simulink model "FIR_32tap_HIL"  (Simulink 7.0)
settings: Solver=FixedStepDiscrete  StartTime=0.0  StopTime=1024*sample_time  RelTol=1e-3
PreLoadFcn:
  | FIR_32tap_setup
InitFcn:
  | %% DSPBuilder Start
  | alt_dspbuilder_update_model(bdroot)
  | %% DSPBuilder End
undefined symbols (not defined in the file): get, sample_time
libraries: allblocks_alteradspbuilder2 x8, dspsnks4 x2, simulink x1
settings Model: Creator=davlin  LastModifiedBy=davlin
settings DebuggingCC: SaveWithParameterizedLinksMsg=none
settings GRTTargetCC: TargetFcnLib=ansi_tfl_tmw.mat

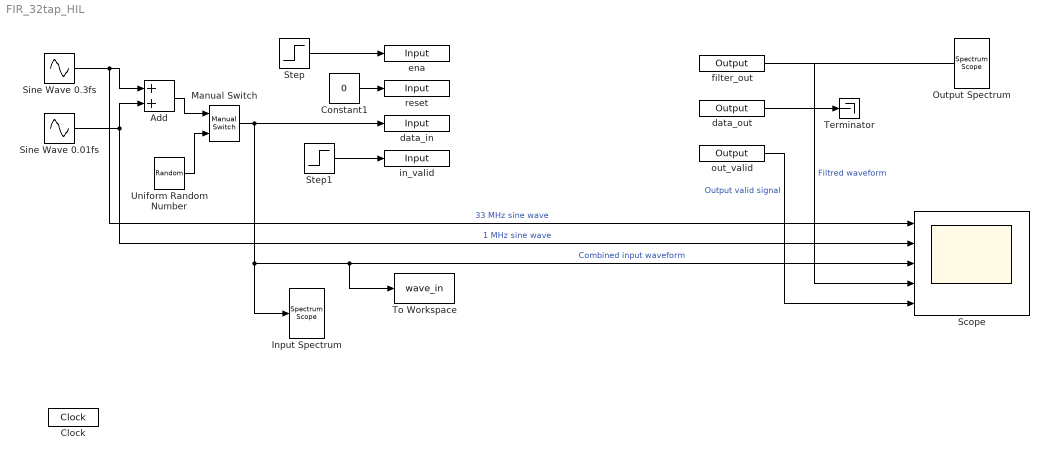
== system FIR_32tap_HIL ==
  Add : Sum  OutDataType=sfix(16)  OutScaling=2^-10
  Clock : allblocks_alteradspbuilder2/Clock  ClockPeriod=clock_period  ClockPeriodUnit=ns  SampleTime=sample_time  SimulationStartCycle=5  PhaseOffset=0  Reset=aclr  ResetType=Active Low  Export=off
  Constant1 : Constant  Value=0  OutDataType=sfix(16)  OutScaling=2^0  SampleTime=sample_time
  Input Spectrum : dspsnks4/Spectrum Scope  DialogController=dspdialog.SpectrumScope  DialogControllerArgs=DataTag0  SystemSampleTime=-1  ScopeProperties=on  Domain=Frequency  HorizSpan=1  UseBuffer=on  BufferSize=128  Overlap=64  inpFftLenInherit=off  FFTlength=128  numAvg=2  DisplayProperties=off  AxisGrid=on  Memory=off  FrameNumber=on  AxisLegend=off  AxisZoom=off  OpenScopeAtSimStart=on  OpenScopeImmediately=off  FigPos=get(0,'defaultfigureposition')  AxisProperties=off  XUnits=Hertz  XRange=[0...Fs/2]  InheritXIncr=on  XIncr=1.0  XLabel=Samples  XLimit=Auto  YUnits=dB  XMax=1  XMin=0  YLabel=Magnitude-squared, dB  LineProperties=off  wintypeSpecScope=Kaiser  RsSpecScope=50  betaSpecScope=5  winsampSpecScope=Periodic
      settings: YMin=7.87541679161896  YMax=68.8425321075722
  Manual Switch : simulink/Signal Routing/Manual Switch  SystemSampleTime=-1  sw=1  action=0  varsize=off
  Output Spectrum : dspsnks4/Spectrum Scope  DialogController=dspdialog.SpectrumScope  DialogControllerArgs=DataTag1  SystemSampleTime=-1  ScopeProperties=on  Domain=Frequency  HorizSpan=1  UseBuffer=on  BufferSize=128  Overlap=64  inpFftLenInherit=off  FFTlength=128  numAvg=2  DisplayProperties=off  AxisGrid=on  Memory=off  FrameNumber=on  AxisLegend=off  AxisZoom=off  OpenScopeAtSimStart=on  OpenScopeImmediately=off  FigPos=get(0,'defaultfigureposition')  AxisProperties=off  XUnits=Hertz  XRange=[0...Fs/2]  InheritXIncr=on  XIncr=1.0  XLabel=Samples  XLimit=Auto  YUnits=dB  XMax=1  XMin=0  YLabel=Magnitude-squared, dB  LineProperties=off  wintypeSpecScope=Kaiser  RsSpecScope=50  betaSpecScope=5  winsampSpecScope=Periodic
      settings: YMin=64.9503892288853  YMax=135.181542756045
  Scope : Scope  NumInputPorts=5
      settings: YMin=-500~-750~-1000~-750~-5  YMax=500~750~1000~750~5  Decimation=sample_time  SampleInput=on  SampleTime=sample_time
  Sine Wave 0.01fs : Sin  SineType=Sample based  Amplitude=2^9-1  Samples=100  SampleTime=sample_time
  Sine Wave 0.3fs : Sin  SineType=Sample based  Amplitude=2^9-1  Samples=3  SampleTime=sample_time
  Step : Step  Time=sample_time  SampleTime=sample_time
  Step1 : Step  Time=sample_time  SampleTime=sample_time
  Terminator : Terminator
  To Workspace : ToWorkspace  VariableName=wave_in  SampleTime=-1  SaveFormat=Array
  Uniform Random Number : UniformRandomNumber  Minimum=-2^10  Maximum=2^10-1  SampleTime=sample_time
  data_in : allblocks_alteradspbuilder2/Input  iofile=C:\Training\DSP_Training\Labs\DSPB_QII_V_9_0\Ex3\partb\tb_FIR_32tap_HIL\FIR%5F32tap%5FHIL_data%5Fin.salt  BusType=Signed Integer  bwl=12  bwr=0  SpecifyClock=on  clock=Clock  PORTTYPE=Input  externalType=Inferred  allowFloatingPointOverride=on  logOutputs=off
  data_out : allblocks_alteradspbuilder2/Output  iofile=C:\Training\DSP_Training\Labs\DSPB_QII_V_9_0\Ex3\partb\tb_FIR_32tap_HIL\FIR%5F32tap%5FHIL_data%5Fout.capture  BusType=Signed Integer  bwl=12  bwr=0  externalType=Inferred  PORTTYPE=Output  allowFloatingPointOverride=on  logOutputs=off
  ena : allblocks_alteradspbuilder2/Input  iofile=C:\Training\DSP_Training\Labs\DSPB_QII_V_9_0\Ex3\partb\tb_FIR_32tap_HIL\FIR%5F32tap%5FHIL_ena.salt  BusType=Single Bit  bwl=8  bwr=0  SpecifyClock=on  clock=Clock  PORTTYPE=Input  externalType=Inferred  allowFloatingPointOverride=on  logOutputs=off
  filter_out : allblocks_alteradspbuilder2/Output  iofile=C:\Training\DSP_Training\Labs\DSPB_QII_V_9_0\Ex3\partb\tb_FIR_32tap_HIL\FIR%5F32tap%5FHIL_filter%5Fout.capture  BusType=Signed Fractional  bwl=16  bwr=11  externalType=Inferred  PORTTYPE=Output  allowFloatingPointOverride=on  logOutputs=off
  in_valid : allblocks_alteradspbuilder2/Input  iofile=C:\Training\DSP_Training\Labs\DSPB_QII_V_9_0\Ex3\partb\tb_FIR_32tap_HIL\FIR%5F32tap%5FHIL_in%5Fvalid.salt  BusType=Single Bit  bwl=8  bwr=0  SpecifyClock=on  clock=Clock  PORTTYPE=Input  externalType=Inferred  allowFloatingPointOverride=on  logOutputs=off
  out_valid : allblocks_alteradspbuilder2/Output  iofile=C:\Training\DSP_Training\Labs\DSPB_QII_V_9_0\Ex3\partb\tb_FIR_32tap_HIL\FIR%5F32tap%5FHIL_out%5Fvalid.capture  BusType=Single Bit  bwl=8  bwr=0  externalType=Inferred  PORTTYPE=Output  allowFloatingPointOverride=on  logOutputs=off
  reset : allblocks_alteradspbuilder2/Input  iofile=C:\Training\DSP_Training\Labs\DSPB_QII_V_9_0\Ex3\partb\tb_FIR_32tap_HIL\FIR%5F32tap%5FHIL_reset.salt  BusType=Single Bit  bwl=8  bwr=0  SpecifyClock=on  clock=Clock  PORTTYPE=Input  externalType=Inferred  allowFloatingPointOverride=on  logOutputs=off
  wires:
  Step/1 -> ena/1
  Constant1/1 -> reset/1
  Step1/1 -> in_valid/1
  filter_out/1 -> Output Spectrum/1, Scope/4  "Filtred waveform"
  Manual Switch/1 -> data_in/1, Input Spectrum/1, Scope/3, To Workspace/1  "Combined input waveform"
  Sine Wave 0.3fs/1 -> Add/1, Scope/1  "33 MHz sine wave"
  Sine Wave 0.01fs/1 -> Add/2, Scope/2  "1 MHz sine wave"
  Uniform Random Number/1 -> Manual Switch/2
  out_valid/1 -> Scope/5  "Output valid signal"
  Add/1 -> Manual Switch/1
  data_out/1 -> Terminator/1
